simulink model "wzorzec"  (R2023b)
settings: Solver=ode5  StartTime=0.0  StopTime=Inf  FixedStep=0.01  RelTol=1e-3
values from neighbouring files (symbols this model uses):
  A = [0 1 0;-4.550992177770367*cos(xr(1)+0.351605023736978) -0.211992177343933+2.179474529348904e-04*abs(xr(3)) 4.571825606174361*dF(xr(3))-sign*2.179474529348904e-04*xr(2);0 0 7.645471000671387e+03*dH(xr(3))]    [get_abcd.m]
  B = [0;0;7.645471000671387e+03]    [get_abcd.m]
  C = [1 0 0;0 0 1]    [get_abcd.m]
  K = p(2)    [cel_00.m]    (also in main.m = lqr(A1,B1,Q1,R1); rhs_02.m = 7645.47100067)
  L = lqe(A,G,C,Q,R)    [main.m]
  ur = 1.28308710741392e-11*x3r.^3-9.47671659934249e-10*x3r.^2+0.000162289932269009*x3r-0.00418773065630636    [get_eqpoint.m]
  xr = [x1r;0;x3r]    [get_eqpoint.m]
settings Model: SimulationMode=external  Creator=STUDENT  LastModifiedBy=kamil
settings SolverCC: AlgebraicLoopSolver=TrustRegion  DecoupledContinuousIntegration=on  MinimalZcImpactIntegration=on
settings DataIOCC: ReturnWorkspaceOutputs=off
settings DebuggingCC: UnconnectedInputMsg=warning  UnconnectedOutputMsg=warning  UnconnectedLineMsg=warning  PregeneratedLibrarySubsystemCodeDiagnostic=none  ArithmeticOperatorsInVariantConditions=warning
settings ModelReferenceCC: EnableRefExpFcnMdlSchedulingChecks=on
settings SFSimCC: SimUseLocalCustomCode=off  CustomCodeUndefinedFunction=UseInterfaceOnly
settings RTWCC: Description=Simulink Desktop Real-Time  SystemTargetFile=sldrt.tlc  TemplateMakefile=sldrt.tmf  RTWUseLocalCustomCode=off  RTWCompilerOptimization=on  DLArmComputeVersion=19.05
settings CodeAppCC: MaxIdLength=95
settings SimulinkDesktopRealTimeCC: TargetPreCompLibLocation=C:\apps\MATLAB\R2021b\toolbox\sldrt\lib\win64

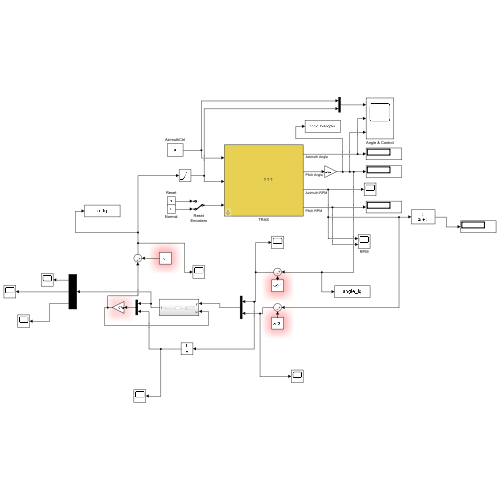
[thumbnail: Simulink's stored preview of the top-level diagram]
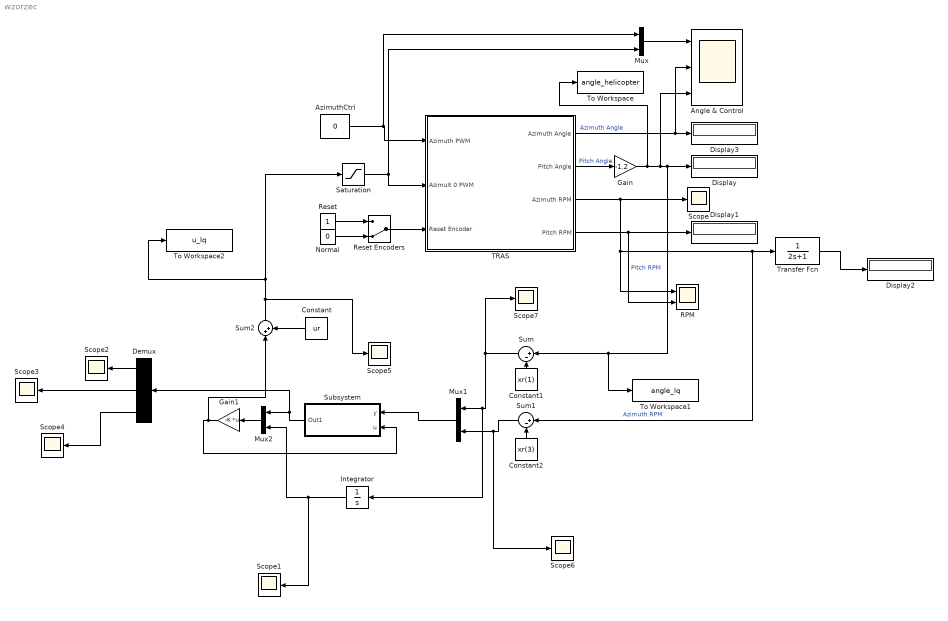
== system wzorzec ==
  Angle & Control : Scope  NumInputPorts=3
  AzimuthCtrl : Constant  Value=0
  Constant : Constant  Value=ur
  Constant1 : Constant  Value=xr(1)
  Constant2 : Constant  Value=xr(3)
  Demux : Demux  Outputs=3
  Display{,1..3} (4 alike) : Display
  Gain : Gain  Gain=-1.2
  Gain1 : Gain  Gain=-K  Multiplication=Matrix(K*u)
  Integrator : Integrator
  Mux : Mux  Inputs=2
  Mux1 : Mux  Inputs=2
  Mux2 : Mux  Inputs=2
  Normal : Constant  Value=0
  RPM : Scope  NumInputPorts=2
  Reset : Constant
  Reset Encoders : ManualSwitch  CurrentSetting=0
  Saturation : Saturate  UpperLimit=0.6  LowerLimit=-0.6
  Scope{,1..7} (8 alike) : Scope
  Subsystem : Subsystem
  Sum : Sum  Inputs=|+-
  Sum1 : Sum  Inputs=|+-
  Sum2 : Sum  Inputs=|++
  TRAS : Subsystem  mask{BaseAddress=57088, T0=0.01}
      mask prompts: BaseAddress "Base Address:"; T0 "Sampling Period:"
      mask Display: image('TRAS.JPG')
  To Workspace : ToWorkspace  VariableName=angle_helicopter  SaveFormat=Structure With Time  SampleTime=0.01
  To Workspace1 : ToWorkspace  VariableName=angle_lq  SaveFormat=Structure With Time  SampleTime=-1
  To Workspace2 : ToWorkspace  VariableName=u_lq  SaveFormat=Structure With Time  SampleTime=-1
  Transfer Fcn : TransferFcn  Denominator=[2 1]
  wires:
  Reset/1 -> Reset Encoders/1
  TRAS/3(Azimuth RPM) -> Scope/1, Sum1/1, Transfer Fcn/1, RPM/1  "Azimuth RPM"
  TRAS/1(Azimuth Angle) -> Angle & Control/2, Display3/1  "Azimuth Angle"
  TRAS/4(Pitch RPM) -> RPM/2, Display1/1  "Pitch RPM"
  Normal/1 -> Reset Encoders/2
  Reset Encoders/1 -> TRAS/3(Reset Encoder)
  TRAS/2(Pitch Angle) -> Gain/1  "Pitch Angle"
  Gain/1 -> To Workspace/1, To Workspace1/1, Sum/1, Display/1, Angle & Control/3
  Mux/1 -> Angle & Control/1
  AzimuthCtrl/1 -> Mux/1, TRAS/1(Azimuth PWM)
  Transfer Fcn/1 -> Display2/1
  Saturation/1 -> TRAS/2(Azimult 0 PWM), Mux/2
  Subsystem/1(Out1) -> Mux2/1, Demux/1
  Mux1/1 -> Subsystem/1(y)
  Constant1/1 -> Sum/2
  Sum/1 -> Scope7/1, Integrator/1, Mux1/1
  Constant2/1 -> Sum1/2
  Sum1/1 -> Scope6/1, Mux1/2
  Demux/1 -> Scope2/1
  Demux/2 -> Scope3/1
  Demux/3 -> Scope4/1
  Sum2/1 -> Saturation/1, To Workspace2/1, Scope5/1
  Constant/1 -> Sum2/2
  Integrator/1 -> Scope1/1, Mux2/2
  Mux2/1 -> Gain1/1
  Gain1/1 -> Sum2/1, Subsystem/2(u)

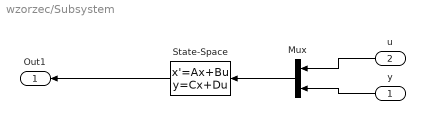
== system wzorzec/Subsystem ==
  y : Inport
  u : Inport  Port=2
  Mux : Mux  Inputs=2
  State-Space : StateSpace  A=A-L*C  B=[B L]  C=eye(3)  D=zeros(3,3)  InitialCondition=zeros(3,1)
  Out1 : Outport
  wires:
  u/1 -> Mux/1
  y/1 -> Mux/2
  Mux/1 -> State-Space/1
  State-Space/1 -> Out1/1

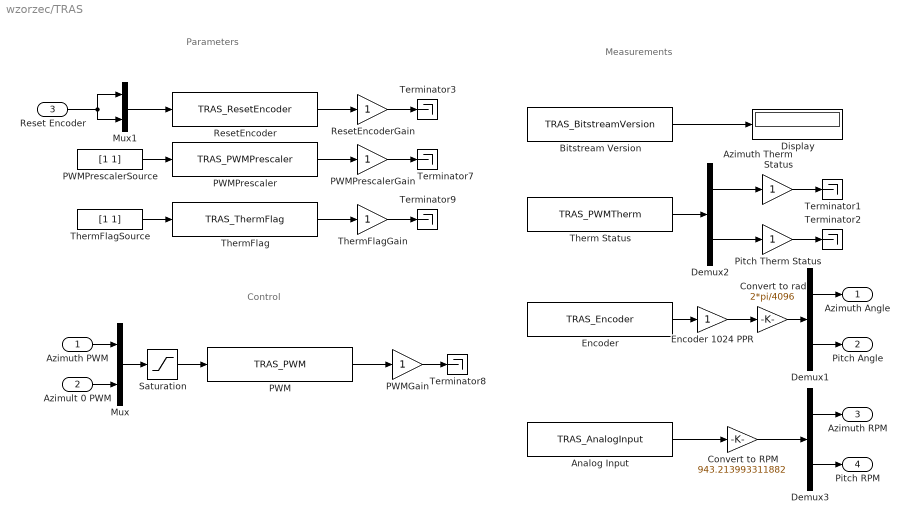
== system wzorzec/TRAS ==
  note: Parameters
  note: Control
  note: Measurements
  Azimuth PWM : Inport
  Azimult 0 PWM : Inport  Port=2
  Reset Encoder : Inport  Port=3
  Analog Input : S-Function  FunctionName=TRAS_AnalogInput  Parameters=BaseAddress, [1 0], [1 1], T0  SFunctionDeploymentMode=off  EnableBusSupport=off
  Azimuth Therm Status : Gain  SaturateOnIntegerOverflow=on  OutDataTypeStr=Inherit: Same as input  ParamDataTypeStr=Inherit: Same as input
  Bitstream Version : S-Function  FunctionName=TRAS_BitstreamVersion  Parameters=BaseAddress, T0  SFunctionDeploymentMode=off  EnableBusSupport=off
  Convert to RPM : Gain  Gain=943.213993311882  SaturateOnIntegerOverflow=on  OutDataTypeStr=Inherit: Same as input  ParamDataTypeStr=Inherit: Same as input
  Convert to rad : Gain  Gain=2*pi/4096  SaturateOnIntegerOverflow=on  OutDataTypeStr=Inherit: Same as input  ParamDataTypeStr=Inherit: Same as input
  Demux1 : Demux  Outputs=2
      settings: DisplayOption=none
  Demux2 : Demux  Outputs=2
      settings: DisplayOption=none
  Demux3 : Demux  Outputs=2
      settings: DisplayOption=none
  Display : Display
  Encoder : S-Function  FunctionName=TRAS_Encoder  Parameters=BaseAddress, T0  SFunctionDeploymentMode=off  EnableBusSupport=off
  Encoder 1024 PPR : Gain  SaturateOnIntegerOverflow=on  OutDataTypeStr=Inherit: Same as input  ParamDataTypeStr=Inherit: Same as input
  Mux : Mux  Inputs=2
  Mux1 : Mux  Inputs=2
  PWM : S-Function  FunctionName=TRAS_PWM  Parameters=BaseAddress, T0  SFunctionDeploymentMode=off  EnableBusSupport=off
  PWMGain : Gain  SaturateOnIntegerOverflow=on  OutDataTypeStr=Inherit: Same as input  ParamDataTypeStr=Inherit: Same as input
  PWMPrescaler : S-Function  FunctionName=TRAS_PWMPrescaler  Parameters=BaseAddress, T0  SFunctionDeploymentMode=off  EnableBusSupport=off
  PWMPrescalerGain : Gain  SaturateOnIntegerOverflow=on  OutDataTypeStr=Inherit: Same as input  ParamDataTypeStr=Inherit: Same as input
  PWMPrescalerSource : Constant  Value=[1 1]
  Pitch Therm Status : Gain  SaturateOnIntegerOverflow=on  OutDataTypeStr=Inherit: Same as input  ParamDataTypeStr=Inherit: Same as input
  ResetEncoder : S-Function  FunctionName=TRAS_ResetEncoder  Parameters=BaseAddress, T0  SFunctionDeploymentMode=off  EnableBusSupport=off
  ResetEncoderGain : Gain  SaturateOnIntegerOverflow=on  OutDataTypeStr=Inherit: Same as input  ParamDataTypeStr=Inherit: Same as input
  Saturation : Saturate  UpperLimit=1  LowerLimit=-1
  Terminator{1..3,7..9} (6 alike) : Terminator
  Therm Status : S-Function  FunctionName=TRAS_PWMTherm  Parameters=BaseAddress, T0  SFunctionDeploymentMode=off  EnableBusSupport=off
  "ThermFlag " : S-Function  FunctionName=TRAS_ThermFlag  Parameters=BaseAddress, T0  SFunctionDeploymentMode=off  EnableBusSupport=off
  ThermFlagGain : Gain  SaturateOnIntegerOverflow=on  OutDataTypeStr=Inherit: Same as input  ParamDataTypeStr=Inherit: Same as input
  ThermFlagSource : Constant  Value=[1 1]
  Azimuth Angle : Outport  VectorParamsAs1DForOutWhenUnconnected=off
  Pitch Angle : Outport  Port=2  VectorParamsAs1DForOutWhenUnconnected=off
  Azimuth RPM : Outport  Port=3  VectorParamsAs1DForOutWhenUnconnected=off
  Pitch RPM : Outport  Port=4  VectorParamsAs1DForOutWhenUnconnected=off
  wires:
  Encoder 1024 PPR/1 -> Convert to rad/1
  Encoder/1 -> Encoder 1024 PPR/1
  Saturation/1 -> PWM/1
  Mux/1 -> Saturation/1
  PWM/1 -> PWMGain/1
  PWMGain/1 -> Terminator8/1
  ResetEncoder/1 -> ResetEncoderGain/1
  PWMPrescaler/1 -> PWMPrescalerGain/1
  Mux1/1 -> ResetEncoder/1
  PWMPrescalerSource/1 -> PWMPrescaler/1
  ResetEncoderGain/1 -> Terminator3/1
  PWMPrescalerGain/1 -> Terminator7/1
  Azimult 0 PWM/1 -> Mux/2
  Azimuth PWM/1 -> Mux/1
  Demux1/2 -> Pitch Angle/1
  Convert to rad/1 -> Demux1/1
  Demux1/1 -> Azimuth Angle/1
  Therm Status/1 -> Demux2/1
  Demux2/2 -> Pitch Therm Status/1
  Demux2/1 -> Azimuth Therm Status/1
  Azimuth Therm Status/1 -> Terminator1/1
  Pitch Therm Status/1 -> Terminator2/1
  Bitstream Version/1 -> Display/1
  Analog Input/1 -> Convert to RPM/1
  Demux3/2 -> Pitch RPM/1
  Demux3/1 -> Azimuth RPM/1
  Reset Encoder/1 -> Mux1/1, Mux1/2
  Convert to RPM/1 -> Demux3/1
  "ThermFlag "/1 -> ThermFlagGain/1
  ThermFlagSource/1 -> "ThermFlag "/1
  ThermFlagGain/1 -> Terminator9/1
